simulink model "CollaborativeErgonomyControl"  (R2021b)
settings: Solver=FixedStepAuto  StartTime=0.0  StopTime=Config.SIMULATION_TIME  FixedStep=Config.tStep  RelTol=1e-3
InitFcn:
  | %% initialize the simulation
  | cd(fileparts(which(bdroot)));
  | initCollaborativeErgonomyControl;
StopFcn:
  | %% stop the simulation
  | cd(fileparts(which(bdroot)));
  | stopCollaborativeErgonomyControl;
values from neighbouring files (symbols this model uses):
  ConfigRobot1 = ConfigRobot    [initCollaborativeErgonomyControl.m]
  ConfigRobot2 = ConfigRobot    [initCollaborativeErgonomyControl.m]
undefined symbols (not defined in the file or in its folder): Config, ConfigObject
libraries: RobotStateLibrary x61, WBToolboxLibrary x40, MultiBodyLibrary x4, simulink x3
(part 1 of 2)
settings Model: NumberOfSteps=100  Creator=lorenzorapetti  LastModifiedBy=icub
settings SolverCC: AlgebraicLoopSolver=TrustRegion
settings DebuggingCC: SFMachineParentedDataDiag=warning

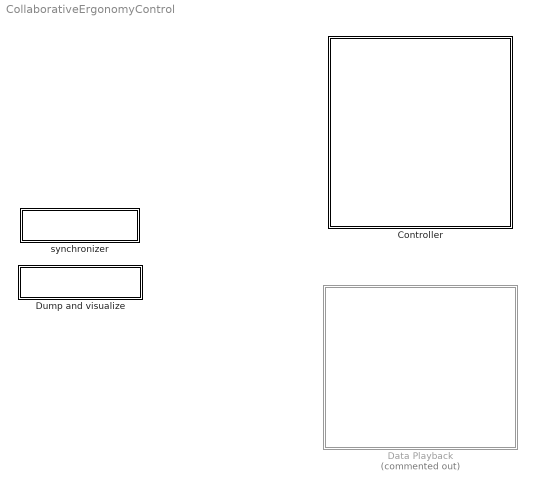
== system CollaborativeErgonomyControl ==
  Controller : Subsystem
  Data Playback : Subsystem  Commented=on
  Dump and visualize : Subsystem
      mask Display: disp('VISUALIZER')
  synchronizer : Subsystem
      mask Display: disp('SYNCHRONIZER')

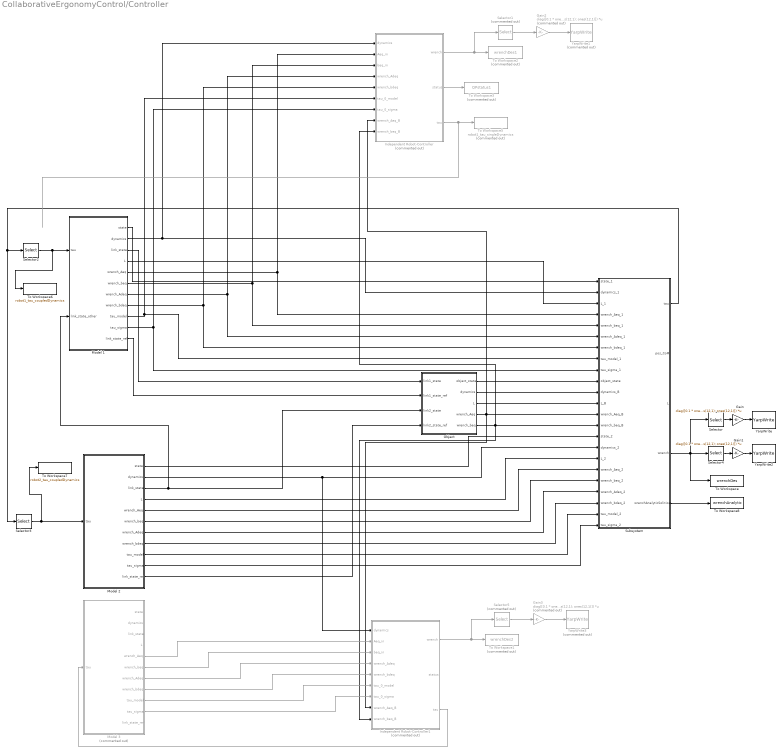
== system CollaborativeErgonomyControl/Controller ==
  Gain : Gain  Gain=diag([0.1 * ones(12,1); ones(12,1)])  Multiplication=Matrix(K*u) (u vector)
  Gain1 : Gain  Gain=diag([0.1 * ones(12,1); ones(12,1)])  Multiplication=Matrix(K*u) (u vector)
  Gain2 : Gain  Commented=on  Gain=diag([0.1 * ones(12,1); ones(12,1)])  Multiplication=Matrix(K*u) (u vector)
  Gain3 : Gain  Commented=on  Gain=diag([0.1 * ones(12,1); ones(12,1)])  Multiplication=Matrix(K*u) (u vector)
  Independent Robot-Controller : Subsystem  Commented=on
  Independent Robot-Controller1 : Subsystem  Commented=on
  Model 1 : Subsystem
  Model 2 : Subsystem
  Model 3 : Subsystem  Commented=on
  Object : Subsystem
  Selector : Selector  IndexOptions=Starting index (dialog)  Indices=1  OutputSizes=24
  Selector1 : Selector  Commented=on  IndexOptions=Starting index (dialog)  Indices=1  OutputSizes=24
  Selector2 : Selector  IndexOptions=Starting index (dialog)  Indices=1  OutputSizes=ConfigRobot1.ROBOT_DOF
  Selector3 : Selector  IndexOptions=Starting index (dialog)  Indices=1+ConfigRobot1.ROBOT_DOF  OutputSizes=ConfigRobot2.ROBOT_DOF
  Selector4 : Selector  IndexOptions=Starting index (dialog)  Indices=25  OutputSizes=24
  Selector5 : Selector  Commented=on  IndexOptions=Starting index (dialog)  Indices=1  OutputSizes=24
  Subsystem : Subsystem
  To Workspace : ToWorkspace  VariableName=wrenchDes  SaveFormat=Timeseries  SampleTime=-1
  To Workspace1 : ToWorkspace  Commented=on  VariableName=wrenchDes2  SaveFormat=Timeseries  SampleTime=-1
  To Workspace2 : ToWorkspace  Commented=on  VariableName=wrenchDes1  SaveFormat=Timeseries  SampleTime=-1
  To Workspace3 : ToWorkspace  Commented=on  VariableName=QPstatus1  SaveFormat=Timeseries  SampleTime=-1
  To Workspace5 : ToWorkspace  Commented=on  VariableName=robot1_tau_singleDynamics  SaveFormat=Timeseries  SampleTime=-1
  To Workspace6 : ToWorkspace  VariableName=robot1_tau_coupledDynamics  SaveFormat=Timeseries  SampleTime=-1
  To Workspace7 : ToWorkspace  VariableName=robot2_tau_coupledDynamics  SaveFormat=Timeseries  SampleTime=-1
  To Workspace8 : ToWorkspace  VariableName=wrenchAnalytic  SaveFormat=Timeseries  SampleTime=-1
  YarpWrite : WBToolboxLibrary/Utilities/YarpWrite  portName='/collaborativeController/robot1/wrench:o'  autoconnect=off  errorOnConnection=on
      settings: SourceProductName=WholeBodyToolbox
  YarpWrite1 : WBToolboxLibrary/Utilities/YarpWrite  Commented=on  portName='/collaborativeController/robot1/singleWrench:o'  autoconnect=off  errorOnConnection=on
      settings: SourceProductName=WholeBodyToolbox
  YarpWrite2 : WBToolboxLibrary/Utilities/YarpWrite  portName='/collaborativeController/robot2/wrench:o'  autoconnect=off  errorOnConnection=on
      settings: SourceProductName=WholeBodyToolbox
  YarpWrite3 : WBToolboxLibrary/Utilities/YarpWrite  Commented=on  portName='/collaborativeController/robot2/singleWrench:o'  autoconnect=off  errorOnConnection=on
      settings: SourceProductName=WholeBodyToolbox
  wires:
  Model 1/11(link_state_ref) -> Object/2(link1_state_ref)
  Object/2(dynamics) -> Subsystem/11(dynamics_B)
  Object/1(object_state) -> Subsystem/10(object_state)
  Model 2/1(state) -> Subsystem/15(state_2)
  Model 1/8(wrench_bdeq) -> Independent Robot-Controller/5(wrench_bdeq), Subsystem/7(wrench_bdeq_1)
  Model 1/2(dynamics) -> Independent Robot-Controller/1(dynamics), Subsystem/2(dynamics_1)
  Model 2/11(link_state_ref) -> Object/4(link2_state_ref)
  Subsystem/1(tau) -> Selector3/1, Selector2/1
  Model 2/10(tau_sigma) -> Subsystem/23(tau_sigma_2)
  Model 1/1(state) -> Subsystem/1(state_1)
  Model 2/4(L) -> Subsystem/17(L_2)
  Object/5(wrench_beq) -> Independent Robot-Controller1/9(wrench_beq_B), Independent Robot-Controller/9(wrench_beq_B), Subsystem/14(wrench_beq_B)
  Model 1/4(L) -> Subsystem/3(L_1)
  Model 2/2(dynamics) -> Independent Robot-Controller1/1(dynamics), Subsystem/16(dynamics_2)
  Model 2/9(tau_model) -> Subsystem/22(tau_model_2)
  Model 2/6(wrench_beq) -> Subsystem/19(wrench_beq_2)
  Object/4(wrench_Aeq) -> Independent Robot-Controller1/8(wrench_Aeq_B), Independent Robot-Controller/8(wrench_Aeq_B), Subsystem/13(wrench_Aeq_B)
  Model 2/3(link_state) -> Model 1/2(link_state_other), Object/3(link2_state)
  Model 2/5(wrench_Aeq) -> Subsystem/18(wrench_Aeq_2)
  Model 2/7(wrench_Adeq) -> Subsystem/20(wrench_Adeq_2)
  Independent Robot-Controller/2(status) -> To Workspace3/1
  Model 1/3(link_state) -> Object/1(link1_state)
  Model 1/10(tau_sigma) -> Independent Robot-Controller/7(tau_0_sigma), Subsystem/9(tau_sigma_1)
  Model 2/8(wrench_bdeq) -> Subsystem/21(wrench_bdeq_2)
  Model 1/5(wrench_Aeq) -> Independent Robot-Controller/2(Aeq_in), Subsystem/4(wrench_Aeq_1)
  Model 1/7(wrench_Adeq) -> Independent Robot-Controller/4(wrench_Adeq), Subsystem/6(wrench_Adeq_1)
  Object/3(L) -> Subsystem/12(L_B)
  Model 1/6(wrench_beq) -> Independent Robot-Controller/3(beq_in), Subsystem/5(wrench_beq_1)
  Model 1/9(tau_model) -> Independent Robot-Controller/6(tau_0_model), Subsystem/8(tau_model_1)
  Independent Robot-Controller1/3(tau) -> Model 3/1(tau)
  Selector3/1 -> To Workspace7/1, Model 2/1(tau)
  Model 3/5(wrench_Aeq) -> Independent Robot-Controller1/2(Aeq_in)
  Model 3/6(wrench_beq) -> Independent Robot-Controller1/3(beq_in)
  Model 3/7(wrench_Adeq) -> Independent Robot-Controller1/4(wrench_Adeq)
  Model 3/8(wrench_bdeq) -> Independent Robot-Controller1/5(wrench_bdeq)
  Model 3/9(tau_model) -> Independent Robot-Controller1/6(tau_0_model)
  Model 3/10(tau_sigma) -> Independent Robot-Controller1/7(tau_0_sigma)
  Independent Robot-Controller/3(tau) -> To Workspace5/1
  Selector/1 -> Gain/1
  Independent Robot-Controller/1(wrench) -> Selector1/1, To Workspace2/1
  Subsystem/4(wrench) -> Selector4/1, To Workspace/1, Selector/1
  Gain/1 -> YarpWrite/1
  Selector4/1 -> Gain1/1
  Gain1/1 -> YarpWrite2/1
  Gain2/1 -> YarpWrite1/1
  Selector1/1 -> Gain2/1
  Subsystem/5(wrenchAnalyticSolition) -> To Workspace8/1
  Independent Robot-Controller1/1(wrench) -> Selector5/1, To Workspace1/1
  Selector5/1 -> Gain3/1
  Gain3/1 -> YarpWrite3/1
  Selector2/1 -> To Workspace6/1, Model 1/1(tau)

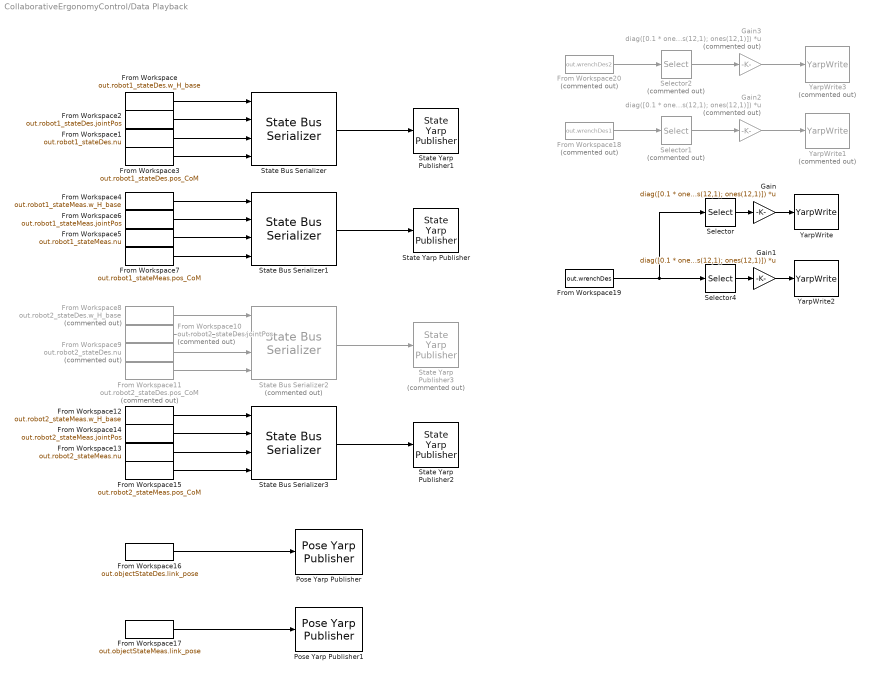
== system CollaborativeErgonomyControl/Data Playback ==
  From Workspace : FromWorkspace  VariableName=out.robot1_stateDes.w_H_base  OutputAfterFinalValue=Holding final value
  From Workspace1 : FromWorkspace  VariableName=out.robot1_stateDes.nu  OutputAfterFinalValue=Holding final value
  From Workspace10 : FromWorkspace  Commented=on  VariableName=out.robot2_stateDes.jointPos  OutputAfterFinalValue=Holding final value
  From Workspace11 : FromWorkspace  Commented=on  VariableName=out.robot2_stateDes.pos_CoM  OutputAfterFinalValue=Holding final value
  From Workspace12 : FromWorkspace  VariableName=out.robot2_stateMeas.w_H_base  OutputAfterFinalValue=Holding final value
  From Workspace13 : FromWorkspace  VariableName=out.robot2_stateMeas.nu  OutputAfterFinalValue=Holding final value
  From Workspace14 : FromWorkspace  VariableName=out.robot2_stateMeas.jointPos  OutputAfterFinalValue=Holding final value
  From Workspace15 : FromWorkspace  VariableName=out.robot2_stateMeas.pos_CoM  OutputAfterFinalValue=Holding final value
  From Workspace16 : FromWorkspace  VariableName=out.objectStateDes.link_pose  OutputAfterFinalValue=Holding final value
  From Workspace17 : FromWorkspace  VariableName=out.objectStateMeas.link_pose  OutputAfterFinalValue=Holding final value
  From Workspace18 : FromWorkspace  Commented=on  VariableName=out.wrenchDes1  OutputAfterFinalValue=Holding final value
  From Workspace19 : FromWorkspace  VariableName=out.wrenchDes  OutputAfterFinalValue=Holding final value
  From Workspace2 : FromWorkspace  VariableName=out.robot1_stateDes.jointPos  OutputAfterFinalValue=Holding final value
  From Workspace20 : FromWorkspace  Commented=on  VariableName=out.wrenchDes2  OutputAfterFinalValue=Holding final value
  From Workspace3 : FromWorkspace  VariableName=out.robot1_stateDes.pos_CoM  OutputAfterFinalValue=Holding final value
  From Workspace4 : FromWorkspace  VariableName=out.robot1_stateMeas.w_H_base  OutputAfterFinalValue=Holding final value
  From Workspace5 : FromWorkspace  VariableName=out.robot1_stateMeas.nu  OutputAfterFinalValue=Holding final value
  From Workspace6 : FromWorkspace  VariableName=out.robot1_stateMeas.jointPos  OutputAfterFinalValue=Holding final value
  From Workspace7 : FromWorkspace  VariableName=out.robot1_stateMeas.pos_CoM  OutputAfterFinalValue=Holding final value
  From Workspace8 : FromWorkspace  Commented=on  VariableName=out.robot2_stateDes.w_H_base  OutputAfterFinalValue=Holding final value
  From Workspace9 : FromWorkspace  Commented=on  VariableName=out.robot2_stateDes.nu  OutputAfterFinalValue=Holding final value
  Gain : Gain  Gain=diag([0.1 * ones(12,1); ones(12,1)])  Multiplication=Matrix(K*u) (u vector)
  Gain1 : Gain  Gain=diag([0.1 * ones(12,1); ones(12,1)])  Multiplication=Matrix(K*u) (u vector)
  Gain2 : Gain  Commented=on  Gain=diag([0.1 * ones(12,1); ones(12,1)])  Multiplication=Matrix(K*u) (u vector)
  Gain3 : Gain  Commented=on  Gain=diag([0.1 * ones(12,1); ones(12,1)])  Multiplication=Matrix(K*u) (u vector)
  Pose Yarp Publisher : RobotStateLibrary/Pose Yarp Publisher  portName='/collaborativeController/boxRef/basePose:o'
      settings: SourceProductName=robot-state-library
  Pose Yarp Publisher1 : RobotStateLibrary/Pose Yarp Publisher  portName='/collaborativeController/box/basePose:o'
      settings: SourceProductName=robot-state-library
  Selector : Selector  IndexOptions=Starting index (dialog)  Indices=1  OutputSizes=24
  Selector1 : Selector  Commented=on  IndexOptions=Starting index (dialog)  Indices=1  OutputSizes=24
  Selector2 : Selector  Commented=on  IndexOptions=Starting index (dialog)  Indices=1  OutputSizes=24
  Selector4 : Selector  IndexOptions=Starting index (dialog)  Indices=25  OutputSizes=24
  State Bus Serializer : RobotStateLibrary/State Bus Serializer  SystemSampleTime=-1  VariantActivationTime=update diagram  Latency=0  AutoFrameSizeCalculation=off
      settings: SourceProductName=robot-state-library
  State Bus Serializer1 : RobotStateLibrary/State Bus Serializer  SystemSampleTime=-1  VariantActivationTime=update diagram  Latency=0  AutoFrameSizeCalculation=off
      settings: SourceProductName=robot-state-library
  State Bus Serializer2 : RobotStateLibrary/State Bus Serializer  Commented=on  SystemSampleTime=-1  VariantActivationTime=update diagram  Latency=0  AutoFrameSizeCalculation=off
      settings: SourceProductName=robot-state-library
  State Bus Serializer3 : RobotStateLibrary/State Bus Serializer  SystemSampleTime=-1  VariantActivationTime=update diagram  Latency=0  AutoFrameSizeCalculation=off
      settings: SourceProductName=robot-state-library
  State Yarp Publisher : RobotStateLibrary/State Yarp Publisher  basePosePortName='/collaborativeController/robot1/basePose:o'  jointPosPortName='/collaborativeController/robot1/jointPosition:o'  nuPortName='/collaborativeController/robot1/stateVelocity:o'  posCoMPortName='/collaborativeController/robot1/CoMPosition:o'
      settings: SourceProductName=robot-state-library
  State Yarp Publisher1 : RobotStateLibrary/State Yarp Publisher  basePosePortName='/collaborativeController/robot1Ref/basePose:o'  jointPosPortName='/collaborativeController/robot1Ref/jointPosition:o'  nuPortName='/collaborativeController/robot1Ref/stateVelocity:o'  posCoMPortName='/collaborativeController/robot1Ref/CoMPosition:o'
      settings: SourceProductName=robot-state-library
  State Yarp Publisher2 : RobotStateLibrary/State Yarp Publisher  basePosePortName='/collaborativeController/robot2/basePose:o'  jointPosPortName='/collaborativeController/robot2/jointPosition:o'  nuPortName='/collaborativeController/robot2/stateVelocity:o'  posCoMPortName='/collaborativeController/robot2/CoMPosition:o'
      settings: SourceProductName=robot-state-library
  State Yarp Publisher3 : RobotStateLibrary/State Yarp Publisher  Commented=on  basePosePortName='/collaborativeController/robot2Ref/basePose:o'  jointPosPortName='/collaborativeController/robot2Ref/jointPosition:o'  nuPortName='/collaborativeController/robot2Ref/stateVelocity:o'  posCoMPortName='/collaborativeController/robot2Ref/CoMPosition:o'
      settings: SourceProductName=robot-state-library
  YarpWrite : WBToolboxLibrary/Utilities/YarpWrite  portName='/collaborativeController/robot1/wrench:o'  autoconnect=off  errorOnConnection=on
      settings: SourceProductName=WholeBodyToolbox
  YarpWrite1 : WBToolboxLibrary/Utilities/YarpWrite  Commented=on  portName='/collaborativeController/robot1/singleWrench:o'  autoconnect=off  errorOnConnection=on
      settings: SourceProductName=WholeBodyToolbox
  YarpWrite2 : WBToolboxLibrary/Utilities/YarpWrite  portName='/collaborativeController/robot2/wrench:o'  autoconnect=off  errorOnConnection=on
      settings: SourceProductName=WholeBodyToolbox
  YarpWrite3 : WBToolboxLibrary/Utilities/YarpWrite  Commented=on  portName='/collaborativeController/robot2/singleWrench:o'  autoconnect=off  errorOnConnection=on
      settings: SourceProductName=WholeBodyToolbox
  wires:
  From Workspace3/1 -> State Bus Serializer/4
  State Bus Serializer/1 -> State Yarp Publisher1/1
  From Workspace2/1 -> State Bus Serializer/2
  From Workspace4/1 -> State Bus Serializer1/1
  From Workspace7/1 -> State Bus Serializer1/4
  From Workspace1/1 -> State Bus Serializer/3
  From Workspace6/1 -> State Bus Serializer1/2
  State Bus Serializer1/1 -> State Yarp Publisher/1
  From Workspace5/1 -> State Bus Serializer1/3
  From Workspace/1 -> State Bus Serializer/1
  From Workspace15/1 -> State Bus Serializer3/4
  From Workspace12/1 -> State Bus Serializer3/1
  State Bus Serializer2/1 -> State Yarp Publisher3/1
  From Workspace8/1 -> State Bus Serializer2/1
  From Workspace14/1 -> State Bus Serializer3/2
  From Workspace10/1 -> State Bus Serializer2/2
  State Bus Serializer3/1 -> State Yarp Publisher2/1
  From Workspace11/1 -> State Bus Serializer2/4
  From Workspace13/1 -> State Bus Serializer3/3
  From Workspace9/1 -> State Bus Serializer2/3
  From Workspace16/1 -> Pose Yarp Publisher/1
  From Workspace17/1 -> Pose Yarp Publisher1/1
  Gain2/1 -> YarpWrite1/1
  Selector1/1 -> Gain2/1
  From Workspace18/1 -> Selector1/1
  Gain1/1 -> YarpWrite2/1
  Selector/1 -> Gain/1
  From Workspace19/1 -> Selector4/1, Selector/1
  Selector4/1 -> Gain1/1
  Gain/1 -> YarpWrite/1
  From Workspace20/1 -> Selector2/1
  Gain3/1 -> YarpWrite3/1
  Selector2/1 -> Gain3/1

== system CollaborativeErgonomyControl/Dump and visualize ==
  Clock : Clock
  TIME_SCOPE : Constant  Value=Config.Scopes.TIME_SCOPE
  Time Scope : Subsystem
  wires:
  TIME_SCOPE/1 -> Time Scope/Enable
  [yarp_time] -> Time Scope/1(yarp_time)
  Clock/1 -> Time Scope/2(simulink_time)

== system CollaborativeErgonomyControl/synchronizer ==
  GAZEBO_SYNCHRONIZER : Subsystem
  Logical Operator : Logic  Operator=NOT  AllPortsSameDT=off  OutDataTypeStr=boolean
  "ON_GAZEBO " : Constant  Value=Config.ON_GAZEBO
  REAL_TIME_SYNC : Subsystem
  To Workspace : ToWorkspace  VariableName=yarp_time  SaveFormat=Structure With Time  SampleTime=-1
  Yarp Clock : WBToolboxLibrary/Utilities/Yarp Clock
      settings: SourceProductName=WholeBodyToolbox
  tag scope: yarp_time=global
  wires:
  Logical Operator/1 -> REAL_TIME_SYNC/Enable
  "ON_GAZEBO "/1 -> GAZEBO_SYNCHRONIZER/Enable, Logical Operator/1
  Yarp Clock/1 -> [yarp_time], To Workspace/1

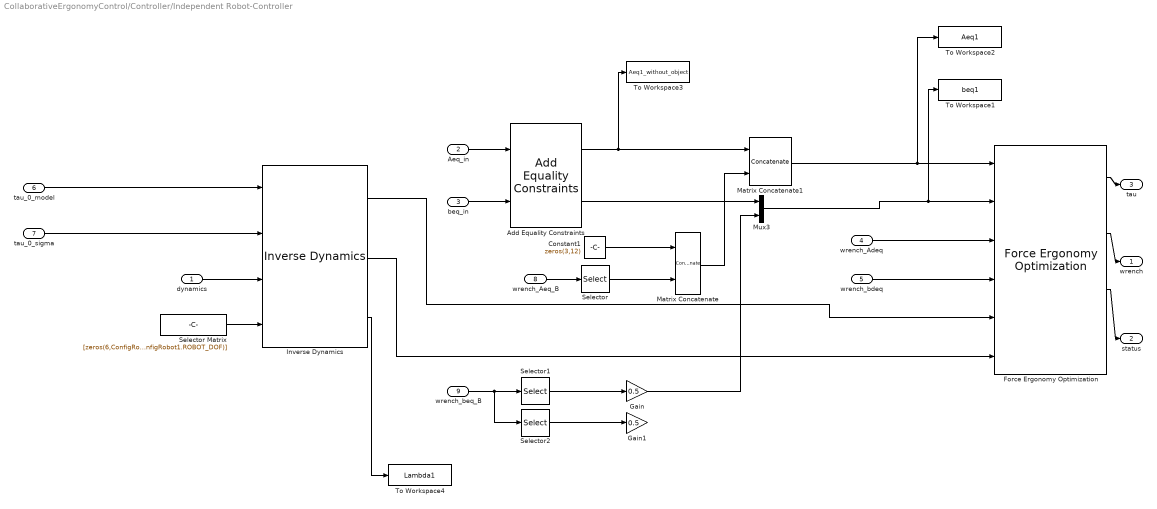
== system CollaborativeErgonomyControl/Controller/Independent Robot-Controller ==
  dynamics : Inport
  Aeq_in : Inport  Port=2
  beq_in : Inport  Port=3
  wrench_Adeq : Inport  Port=4
  wrench_bdeq : Inport  Port=5
  tau_0_model : Inport  Port=6
  tau_0_sigma : Inport  Port=7
  wrench_Aeq_B : Inport  Port=8
  wrench_beq_B : Inport  Port=9
  Add Equality Constraints : RobotStateLibrary/Add Equality Constraints  Aeq_add=ConfigRobot1.wrench_Aeq_const  beq_add=ConfigRobot1.wrench_beq_const
      settings: SourceProductName=robot-state-library
  Constant1 : Constant  Value=zeros(3,12)
  Force Ergonomy Optimization : RobotStateLibrary/Force Ergonomy Optimization  InvTol=ConfigRobot1.Reg.AInvTol  regularizationHessian=ConfigRobot1.Reg.Hessian  minimizationWeight=ConfigRobot1.Gains.tauMinimization
      settings: SourceProductName=robot-state-library
  Gain : Gain  Gain=0.5
  Gain1 : Gain  Gain=0.5
  Inverse Dynamics : RobotStateLibrary/Inverse Dynamics  Reg=ConfigRobot1.Reg  fixedLinkVelcityComponents=ConfigRobot1.fixedLinkVelcityComponents
      settings: SourceProductName=robot-state-library
  Matrix Concatenate : Concatenate  Mode=Multidimensional array  ConcatenateDimension=2
  Matrix Concatenate1 : Concatenate  Mode=Multidimensional array
  Mux3 : Mux  Inputs=2
  Selector : Selector  NumberOfDimensions=2  InputPortWidth=3  IndexOptions=Starting index (dialog),Starting index (dialog)  Indices=1,1  OutputSizes=3,12
  Selector Matrix : Constant  Value=[zeros(6,ConfigRobot1.ROBOT_DOF); eye(ConfigRobot1.ROBOT_DOF)]
  Selector1 : Selector  InputPortWidth=6  IndexOptions=Starting index (dialog)  Indices=1  OutputSizes=3
  Selector2 : Selector  InputPortWidth=6  IndexOptions=Starting index (dialog)  Indices=4  OutputSizes=3
  To Workspace1 : ToWorkspace  VariableName=beq1  SaveFormat=Timeseries  SampleTime=-1
  To Workspace2 : ToWorkspace  VariableName=Aeq1  SaveFormat=Timeseries  SampleTime=-1
  To Workspace3 : ToWorkspace  VariableName=Aeq1_without_object  SaveFormat=Timeseries  SampleTime=-1
  To Workspace4 : ToWorkspace  VariableName=Lambda1  SaveFormat=Timeseries  SampleTime=-1
  wrench : Outport
  status : Outport  Port=2
  tau : Outport  Port=3
  wires:
  wrench_Aeq_B/1 -> Selector/1
  Add Equality Constraints/2 -> Mux3/1
  Constant1/1 -> Matrix Concatenate/1
  wrench_bdeq/1 -> Force Ergonomy Optimization/4
  dynamics/1 -> Inverse Dynamics/3
  Inverse Dynamics/2 -> Force Ergonomy Optimization/6
  wrench_Adeq/1 -> Force Ergonomy Optimization/3
  tau_0_sigma/1 -> Inverse Dynamics/2
  Inverse Dynamics/1 -> Force Ergonomy Optimization/5
  Aeq_in/1 -> Add Equality Constraints/1
  beq_in/1 -> Add Equality Constraints/2
  Force Ergonomy Optimization/3 -> status/1
  Selector/1 -> Matrix Concatenate/2
  Gain/1 -> Mux3/2
  Matrix Concatenate/1 -> Matrix Concatenate1/2
  tau_0_model/1 -> Inverse Dynamics/1
  Force Ergonomy Optimization/2 -> wrench/1
  Force Ergonomy Optimization/1 -> tau/1
  Selector Matrix/1 -> Inverse Dynamics/4
  Add Equality Constraints/1 -> To Workspace3/1, Matrix Concatenate1/1
  wrench_beq_B/1 -> Selector2/1, Selector1/1
  Selector1/1 -> Gain/1
  Selector2/1 -> Gain1/1
  Matrix Concatenate1/1 -> To Workspace2/1, Force Ergonomy Optimization/1
  Mux3/1 -> To Workspace1/1, Force Ergonomy Optimization/2
  Inverse Dynamics/3 -> To Workspace4/1

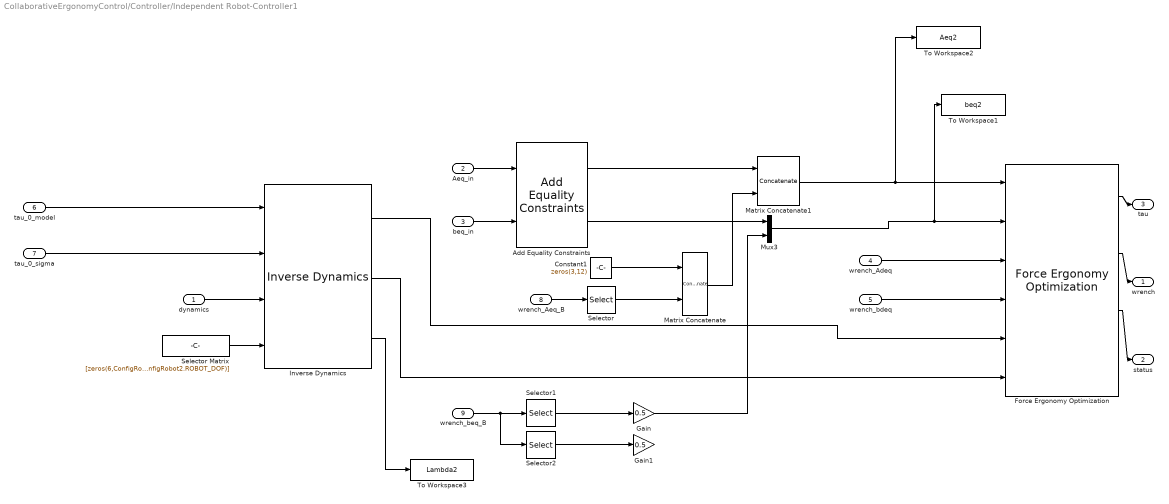
== system CollaborativeErgonomyControl/Controller/Independent Robot-Controller1 ==
  dynamics : Inport
  Aeq_in : Inport  Port=2
  beq_in : Inport  Port=3
  wrench_Adeq : Inport  Port=4
  wrench_bdeq : Inport  Port=5
  tau_0_model : Inport  Port=6
  tau_0_sigma : Inport  Port=7
  wrench_Aeq_B : Inport  Port=8
  wrench_beq_B : Inport  Port=9
  Add Equality Constraints : RobotStateLibrary/Add Equality Constraints  Aeq_add=ConfigRobot2.wrench_Aeq_const  beq_add=ConfigRobot2.wrench_beq_const
      settings: SourceProductName=robot-state-library
  Constant1 : Constant  Value=zeros(3,12)
  Force Ergonomy Optimization : RobotStateLibrary/Force Ergonomy Optimization  InvTol=ConfigRobot2.Reg.AInvTol  regularizationHessian=ConfigRobot2.Reg.Hessian  minimizationWeight=ConfigRobot2.Gains.tauMinimization
      settings: SourceProductName=robot-state-library
  Gain : Gain  Gain=0.5
  Gain1 : Gain  Gain=0.5
  Inverse Dynamics : RobotStateLibrary/Inverse Dynamics  Reg=ConfigRobot2.Reg  fixedLinkVelcityComponents=ConfigRobot2.fixedLinkVelcityComponents
      settings: SourceProductName=robot-state-library
  Matrix Concatenate : Concatenate  Mode=Multidimensional array  ConcatenateDimension=2
  Matrix Concatenate1 : Concatenate  Mode=Multidimensional array
  Mux3 : Mux  Inputs=2
  Selector : Selector  NumberOfDimensions=2  InputPortWidth=3  IndexOptions=Starting index (dialog),Starting index (dialog)  Indices=1,13  OutputSizes=3,12
  Selector Matrix : Constant  Value=[zeros(6,ConfigRobot2.ROBOT_DOF); eye(ConfigRobot2.ROBOT_DOF)]
  Selector1 : Selector  InputPortWidth=6  IndexOptions=Starting index (dialog)  Indices=1  OutputSizes=3
  Selector2 : Selector  InputPortWidth=6  IndexOptions=Starting index (dialog)  Indices=4  OutputSizes=3
  To Workspace1 : ToWorkspace  VariableName=beq2  SaveFormat=Timeseries  SampleTime=-1
  To Workspace2 : ToWorkspace  VariableName=Aeq2  SaveFormat=Timeseries  SampleTime=-1
  To Workspace3 : ToWorkspace  VariableName=Lambda2  SaveFormat=Timeseries  SampleTime=-1
  wrench : Outport
  status : Outport  Port=2
  tau : Outport  Port=3
  wires:
  wrench_Aeq_B/1 -> Selector/1
  Add Equality Constraints/2 -> Mux3/1
  Constant1/1 -> Matrix Concatenate/1
  wrench_bdeq/1 -> Force Ergonomy Optimization/4
  dynamics/1 -> Inverse Dynamics/3
  Inverse Dynamics/2 -> Force Ergonomy Optimization/6
  wrench_Adeq/1 -> Force Ergonomy Optimization/3
  tau_0_sigma/1 -> Inverse Dynamics/2
  Inverse Dynamics/1 -> Force Ergonomy Optimization/5
  Aeq_in/1 -> Add Equality Constraints/1
  beq_in/1 -> Add Equality Constraints/2
  Force Ergonomy Optimization/3 -> status/1
  Selector/1 -> Matrix Concatenate/2
  Gain/1 -> Mux3/2
  Matrix Concatenate/1 -> Matrix Concatenate1/2
  tau_0_model/1 -> Inverse Dynamics/1
  Force Ergonomy Optimization/2 -> wrench/1
  Force Ergonomy Optimization/1 -> tau/1
  Selector Matrix/1 -> Inverse Dynamics/4
  Add Equality Constraints/1 -> Matrix Concatenate1/1
  wrench_beq_B/1 -> Selector2/1, Selector1/1
  Selector1/1 -> Gain/1
  Selector2/1 -> Gain1/1
  Matrix Concatenate1/1 -> To Workspace2/1, Force Ergonomy Optimization/1
  Mux3/1 -> To Workspace1/1, Force Ergonomy Optimization/2
  Inverse Dynamics/3 -> To Workspace3/1

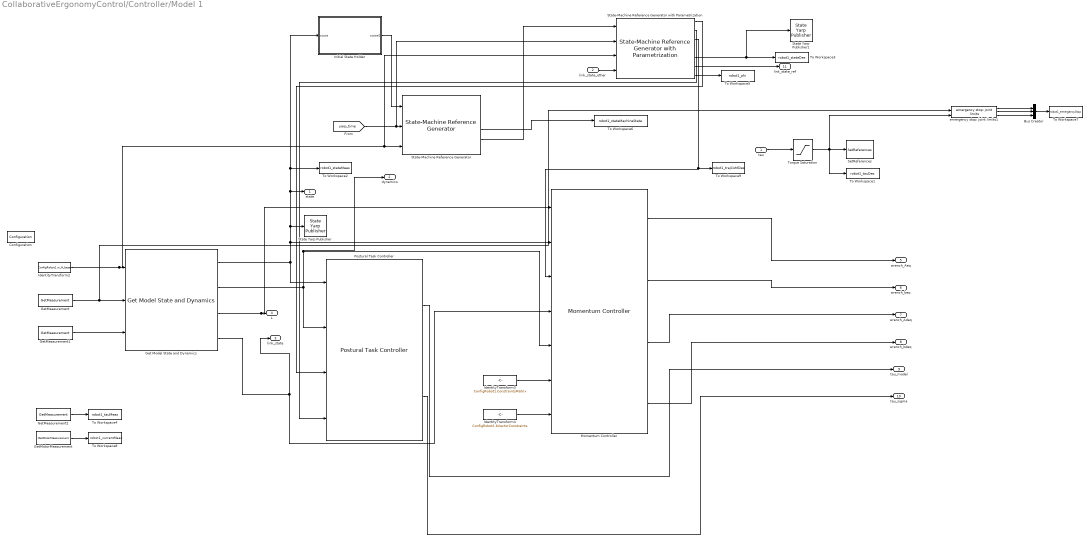
== system CollaborativeErgonomyControl/Controller/Model 1 ==
  tau : Inport
  link_state_other : Inport  Port=2
  Bus Creator : BusCreator  Inputs=3
  Configuration : WBToolboxLibrary/Utilities/Configuration  ConfigSource=Workspace  ConfigObject='WBTConfigRobot_1'
      settings: SourceProductName=WholeBodyToolbox
  Get Model State and Dynamics : RobotStateLibrary/Get Model State and Dynamics  nDoF=ConfigRobot1.ROBOT_DOF  regularization=0.1  contactFrame1Name=ConfigRobot1.Frames.LEFT_FOOT  contactFrame2Name=ConfigRobot1.Frames.RIGHT_FOOT  frame1=ConfigRobot1.Frames.LEFT_FOOT  frame2=ConfigRobot1.Frames.RIGHT_FOOT  frame3=ConfigRobot1.Frames.LEFT_HAND  frame4=ConfigRobot1.Frames.RIGHT_HAND
      settings: SourceProductName=robot-state-library
  GetMeasurement : WBToolboxLibrary/States/GetMeasurement  measuredType=Joints Position
      settings: SourceProductName=WholeBodyToolbox
  GetMeasurement1 : WBToolboxLibrary/States/GetMeasurement  measuredType=Joints Velocity
      settings: SourceProductName=WholeBodyToolbox
  GetMeasurement2 : WBToolboxLibrary/States/GetMeasurement  measuredType=Joints Torque
      settings: SourceProductName=WholeBodyToolbox
  GetMotorMeasurement : WBToolboxLibrary/States/GetMotorMeasurement  measuredType=Motor Current
      settings: SourceProductName=WholeBodyToolbox
  IdentityTransform2 : Constant  Value=ConfigRobot1.w_H_base
  IdentityTransform3 : Constant  Value=ConfigRobot1.ConstraintsMatrix
  IdentityTransform4 : Constant  Value=ConfigRobot1.bVectorConstraints
  Initial State Holder : Subsystem
  Momentum Controller : RobotStateLibrary/Momentum Controller  GainMomentum=ConfigRobot1.Gains.GainMomentum  linksUseConstraintMatrix=ConfigRobot1.linksUseConstraintMatrix
      settings: SourceProductName=robot-state-library
  Postural Task Controller : RobotStateLibrary/Postural Task Controller  GainPostural=ConfigRobot1.Gains.GainPostural
      settings: SourceProductName=robot-state-library
  SetReferences : WBToolboxLibrary/Actuators/SetReferences  controlType=Torque  refSpeed=10*(pi/180)  refAcceleration=1000000*(pi/180)
      settings: SourceProductName=WholeBodyToolbox
  State Yarp Publisher : RobotStateLibrary/State Yarp Publisher  basePosePortName='/collaborativeController/robot1/basePose:o'  jointPosPortName='/collaborativeController/robot1/jointPosition:o'  nuPortName='/collaborativeController/robot1/stateVelocity:o'  posCoMPortName='/collaborativeController/robot1/CoMPosition:o'
      settings: SourceProductName=robot-state-library
  State Yarp Publisher1 : RobotStateLibrary/State Yarp Publisher  basePosePortName='/collaborativeController/robot1Ref/basePose:o'  jointPosPortName='/collaborativeController/robot1Ref/jointPosition:o'  nuPortName='/collaborativeController/robot1Ref/stateVelocity:o'  posCoMPortName='/collaborativeController/robot1Ref/CoMPosition:o'
      settings: SourceProductName=robot-state-library
  State-Machine Reference Generator : RobotStateLibrary/State-Machine Reference Generator  configStateMachine=ConfigRobot1.StateMachine  sampleTime=Config.tStep  frameName1=ConfigRobot1.Frames.LEFT_FOOT  frameName2=ConfigRobot1.Frames.RIGHT_FOOT  regularization=0.1  nDoF=ConfigRobot1.ROBOT_DOF  frame1=ConfigRobot1.Frames.LEFT_FOOT  frame2=ConfigRobot1.Frames.RIGHT_FOOT  frame3=ConfigRobot1.Frames.LEFT_HAND  frame4=ConfigRobot1.Frames.RIGHT_HAND
      settings: SourceProductName=robot-state-library
  State-Machine Reference Generator with Parametrization : RobotStateLibrary/State-Machine Reference Generator with Parametrization  configStateMachine=ConfigRobot1.StateMachine  frameName1=ConfigRobot1.Frames.LEFT_FOOT  frameName2=ConfigRobot1.Frames.RIGHT_FOOT  regularization=0.1  nDoF=ConfigRobot1.ROBOT_DOF  frame1=ConfigRobot1.Frames.LEFT_FOOT  frame2=ConfigRobot1.Frames.RIGHT_FOOT  frame3=ConfigRobot1.Frames.LEFT_HAND  frame4=ConfigRobot1.Frames.RIGHT_HAND  settlingTime=Config.com_minJerk_settlingTime  sampleTime=Config.tStep
      link override Constant: Value=1
      settings: SourceProductName=robot-state-library
  To Workspace1 : ToWorkspace  VariableName=robot1_tauDes  SaveFormat=Timeseries  SampleTime=-1
  To Workspace2 : ToWorkspace  VariableName=robot1_stateMeas  SaveFormat=Timeseries  SampleTime=-1
  To Workspace3 : ToWorkspace  VariableName=robot1_stateDes  SaveFormat=Timeseries  SampleTime=-1
  To Workspace4 : ToWorkspace  VariableName=robot1_tauMeas  SaveFormat=Timeseries  SampleTime=-1
  To Workspace5 : ToWorkspace  VariableName=robot1_phi  SaveFormat=Timeseries  SampleTime=-1
  To Workspace6 : ToWorkspace  VariableName=robot1_stateMachineState  SaveFormat=Timeseries  SampleTime=-1
  To Workspace7 : ToWorkspace  VariableName=robot1_emergencyStop  SaveFormat=Timeseries  SampleTime=-1
  To Workspace8 : ToWorkspace  VariableName=robot1_currentMeas  SaveFormat=Timeseries  SampleTime=-1
  To Workspace9 : ToWorkspace  VariableName=robot1_trajCoMDes  SaveFormat=Timeseries  SampleTime=-1
  Torque Saturation : Saturate  UpperLimit=ConfigRobot1.Safety.torqueSaturation  LowerLimit=-ConfigRobot1.Safety.torqueSaturation
  emergency stop: joint limits1 : RobotStateLibrary/emergency stop: joint limits  Safety=ConfigRobot1.Safety
      settings: SourceProductName=robot-state-library
  state : Outport
  dynamics : Outport  Port=2
  link_state : Outport  Port=3
  L : Outport  Port=4
  wrench_Aeq : Outport  Port=5
  wrench_beq : Outport  Port=6
  wrench_Adeq : Outport  Port=7
  wrench_bdeq : Outport  Port=8
  tau_model : Outport  Port=9
  tau_sigma : Outport  Port=10
  link_state_ref : Outport  Port=11
  wires:
  GetMeasurement/1 -> emergency stop: joint limits1/1, Get Model State and Dynamics/2
  GetMeasurement1/1 -> Get Model State and Dynamics/3
  IdentityTransform2/1 -> State-Machine Reference Generator with Parametrization/3, State-Machine Reference Generator/3, Get Model State and Dynamics/1
  Get Model State and Dynamics/3 -> Momentum Controller/1, L/1
  [yarp_time] -> State-Machine Reference Generator with Parametrization/2, State-Machine Reference Generator/2
  State-Machine Reference Generator/5 -> State-Machine Reference Generator with Parametrization/1
  Get Model State and Dynamics/1 -> Postural Task Controller/1, Momentum Controller/2, To Workspace2/1, Initial State Holder/1(state), state/1, State Yarp Publisher/1
  Initial State Holder/1(state0) -> State-Machine Reference Generator/1
  Get Model State and Dynamics/4 -> link_state/1, Momentum Controller/4
  Get Model State and Dynamics/2 -> Postural Task Controller/2, Momentum Controller/5, dynamics/1
  Momentum Controller/3 -> wrench_Adeq/1
  Momentum Controller/4 -> wrench_bdeq/1
  Postural Task Controller/1 -> tau_model/1
  Postural Task Controller/2 -> tau_sigma/1
  Momentum Controller/1 -> wrench_Aeq/1
  Momentum Controller/2 -> wrench_beq/1
  tau/1 -> Torque Saturation/1
  emergency stop: joint limits1/2 -> Bus Creator/2
  Bus Creator/1 -> To Workspace7/1
  emergency stop: joint limits1/3 -> Bus Creator/3
  emergency stop: joint limits1/1 -> Bus Creator/1
  State-Machine Reference Generator/4 -> To Workspace6/1
  GetMeasurement2/1 -> To Workspace4/1
  Torque Saturation/1 -> emergency stop: joint limits1/2, To Workspace1/1, SetReferences/1
  link_state_other/1 -> State-Machine Reference Generator with Parametrization/4
  State-Machine Reference Generator with Parametrization/1 -> Postural Task Controller/3
  State-Machine Reference Generator with Parametrization/6 -> link_state_ref/1
  State-Machine Reference Generator with Parametrization/7 -> To Workspace5/1
  State-Machine Reference Generator with Parametrization/5 -> To Workspace3/1, State Yarp Publisher1/1
  GetMotorMeasurement/1 -> To Workspace8/1
  State-Machine Reference Generator with Parametrization/2 -> Postural Task Controller/4
  State-Machine Reference Generator with Parametrization/3 -> Momentum Controller/3, To Workspace9/1
  IdentityTransform3/1 -> Momentum Controller/6
  IdentityTransform4/1 -> Momentum Controller/7

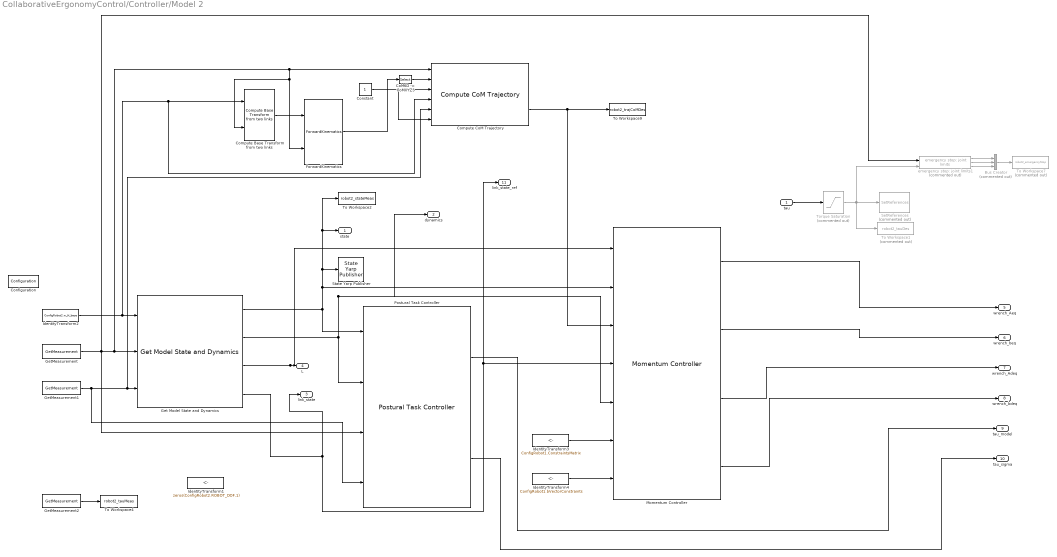
== system CollaborativeErgonomyControl/Controller/Model 2 ==
  tau : Inport
  Bus Creator : BusCreator  Commented=on  Inputs=3
  "CoM6D -> CoMXYZ3" : Selector  NumberOfDimensions=2  InputPortWidth=7  IndexOptions=Index vector (dialog),Index vector (dialog)  Indices=[1 2 3],[4]  OutputSizes=1,1
  Compute Base Transform from two links : RobotStateLibrary/Compute Base Transform from two links  frameName1=ConfigRobot2.Frames.LEFT_FOOT  frameName2=ConfigRobot2.Frames.RIGHT_FOOT
      settings: SourceProductName=robot-state-library
  Compute CoM Trajectory : RobotStateLibrary/Compute CoM Trajectory  frameName1=ConfigRobot2.Frames.LEFT_FOOT  frameName2=ConfigRobot2.Frames.RIGHT_FOOT  regularization=0.1
      settings: SourceProductName=robot-state-library
  Configuration : WBToolboxLibrary/Utilities/Configuration  ConfigSource=Workspace  ConfigObject='WBTConfigRobot_2'
      settings: SourceProductName=WholeBodyToolbox
  Constant : Constant
  ForwardKinematics : WBToolboxLibrary/Model/Kinematics/ForwardKinematics  frameName='com'
      settings: SourceProductName=WholeBodyToolbox
  Get Model State and Dynamics : RobotStateLibrary/Get Model State and Dynamics  nDoF=ConfigRobot2.ROBOT_DOF  regularization=0.1  contactFrame1Name=ConfigRobot2.Frames.LEFT_FOOT  contactFrame2Name=ConfigRobot2.Frames.RIGHT_FOOT  frame1=ConfigRobot2.Frames.LEFT_FOOT  frame2=ConfigRobot2.Frames.RIGHT_FOOT  frame3=ConfigRobot2.Frames.LEFT_HAND  frame4=ConfigRobot2.Frames.RIGHT_HAND
      settings: SourceProductName=robot-state-library
  GetMeasurement : WBToolboxLibrary/States/GetMeasurement  measuredType=Joints Position
      settings: SourceProductName=WholeBodyToolbox
  GetMeasurement1 : WBToolboxLibrary/States/GetMeasurement  measuredType=Joints Velocity
      settings: SourceProductName=WholeBodyToolbox
  GetMeasurement2 : WBToolboxLibrary/States/GetMeasurement  measuredType=Joints Torque
      settings: SourceProductName=WholeBodyToolbox
  IdentityTransform1 : Constant  Value=zeros(ConfigRobot2.ROBOT_DOF,1)
  IdentityTransform2 : Constant  Value=ConfigRobot2.w_H_base
  IdentityTransform3 : Constant  Value=ConfigRobot1.ConstraintsMatrix
  IdentityTransform4 : Constant  Value=ConfigRobot1.bVectorConstraints
  Momentum Controller : RobotStateLibrary/Momentum Controller  GainMomentum=GainMomentumDummy  linksUseConstraintMatrix=ConfigRobot2.linksUseConstraintMatrix
      settings: SourceProductName=robot-state-library
  Postural Task Controller : RobotStateLibrary/Postural Task Controller  GainPostural=GainPosturalDummy
      settings: SourceProductName=robot-state-library
  SetReferences : WBToolboxLibrary/Actuators/SetReferences  Commented=on  controlType=Torque  refSpeed=10*(pi/180)  refAcceleration=1000000*(pi/180)
      settings: SourceProductName=WholeBodyToolbox
  State Yarp Publisher : RobotStateLibrary/State Yarp Publisher  basePosePortName='/collaborativeController/robot2/basePose:o'  jointPosPortName='/collaborativeController/robot2/jointPosition:o'  nuPortName='/collaborativeController/robot2/stateVelocity:o'  posCoMPortName='/collaborativeController/robot2/CoMPosition:o'
      settings: SourceProductName=robot-state-library
  To Workspace1 : ToWorkspace  Commented=on  VariableName=robot2_tauDes  SaveFormat=Timeseries  SampleTime=-1
  To Workspace2 : ToWorkspace  VariableName=robot2_stateMeas  SaveFormat=Timeseries  SampleTime=-1
  To Workspace4 : ToWorkspace  VariableName=robot2_tauMeas  SaveFormat=Timeseries  SampleTime=-1
  To Workspace7 : ToWorkspace  Commented=on  VariableName=robot2_emergencyStop  SaveFormat=Timeseries  SampleTime=-1
  To Workspace9 : ToWorkspace  VariableName=robot2_trajCoMDes  SaveFormat=Timeseries  SampleTime=-1
  Torque Saturation : Saturate  Commented=on  UpperLimit=ConfigRobot2.Safety.torqueSaturation  LowerLimit=-ConfigRobot2.Safety.torqueSaturation
  emergency stop: joint limits1 : RobotStateLibrary/emergency stop: joint limits  Commented=on  Safety=ConfigRobot2.Safety
      settings: SourceProductName=robot-state-library
  state : Outport
  dynamics : Outport  Port=2
  link_state : Outport  Port=3
  L : Outport  Port=4
  wrench_Aeq : Outport  Port=5
  wrench_beq : Outport  Port=6
  wrench_Adeq : Outport  Port=7
  wrench_bdeq : Outport  Port=8
  tau_model : Outport  Port=9
  tau_sigma : Outport  Port=10
  link_state_ref : Outport  Port=11
  wires:
  GetMeasurement1/1 -> Postural Task Controller/4, Compute CoM Trajectory/5, Get Model State and Dynamics/3
  Get Model State and Dynamics/3 -> Momentum Controller/1, L/1
  Get Model State and Dynamics/1 -> Postural Task Controller/1, Momentum Controller/2, To Workspace2/1, state/1, State Yarp Publisher/1
  Get Model State and Dynamics/4 -> link_state/1, Momentum Controller/4, link_state_ref/1
  Get Model State and Dynamics/2 -> Postural Task Controller/2, Momentum Controller/5, dynamics/1
  Momentum Controller/3 -> wrench_Adeq/1
  Momentum Controller/4 -> wrench_bdeq/1
  Postural Task Controller/1 -> tau_model/1
  Postural Task Controller/2 -> tau_sigma/1
  Momentum Controller/1 -> wrench_Aeq/1
  Momentum Controller/2 -> wrench_beq/1
  tau/1 -> Torque Saturation/1
  GetMeasurement2/1 -> To Workspace4/1
  emergency stop: joint limits1/2 -> Bus Creator/2
  Bus Creator/1 -> To Workspace7/1
  emergency stop: joint limits1/3 -> Bus Creator/3
  emergency stop: joint limits1/1 -> Bus Creator/1
  Torque Saturation/1 -> emergency stop: joint limits1/2, To Workspace1/1, SetReferences/1
  Compute Base Transform from two links/1 -> ForwardKinematics/1
  GetMeasurement/1 -> emergency stop: joint limits1/1, Postural Task Controller/3, ForwardKinematics/2, Compute Base Transform from two links/2, Compute CoM Trajectory/1, Get Model State and Dynamics/2
  IdentityTransform2/1 -> Get Model State and Dynamics/1, Compute CoM Trajectory/4, Compute Base Transform from two links/1
  Compute CoM Trajectory/2 -> To Workspace9/1, Momentum Controller/3
  IdentityTransform3/1 -> Momentum Controller/6
  IdentityTransform4/1 -> Momentum Controller/7
  ForwardKinematics/1 -> "CoM6D -> CoMXYZ3"/1
  Constant/1 -> Compute CoM Trajectory/6, Compute CoM Trajectory/3
  "CoM6D -> CoMXYZ3"/1 -> Compute CoM Trajectory/2

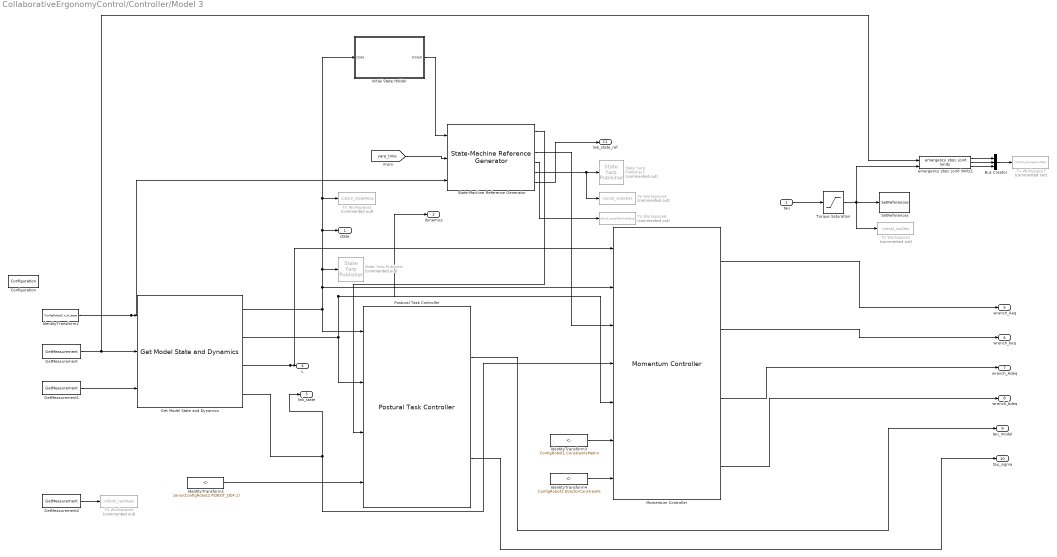
== system CollaborativeErgonomyControl/Controller/Model 3 ==
  tau : Inport
  Bus Creator : BusCreator  Inputs=3
  Configuration : WBToolboxLibrary/Utilities/Configuration  ConfigSource=Workspace  ConfigObject='WBTConfigRobot_2'  RobotName='icubSim'  UrdfFile='model.urdf'  ControlledJoints={'l_elbow','l_shoulder_pitch','torso_roll'}  ControlBoardsNames={'left_arm','right_arm','torso'}  LocalName='WBT'  GravityVector=[0,0,-9.81]
      settings: SourceProductName=WholeBodyToolbox
  Get Model State and Dynamics : RobotStateLibrary/Get Model State and Dynamics  nDoF=ConfigRobot2.ROBOT_DOF  regularization=0.001  contactFrame1Name=ConfigRobot2.Frames.LEFT_FOOT  contactFrame2Name=ConfigRobot2.Frames.RIGHT_FOOT  frame1=ConfigRobot2.Frames.LEFT_FOOT  frame2=ConfigRobot2.Frames.RIGHT_FOOT  frame3=ConfigRobot2.Frames.LEFT_HAND  frame4=ConfigRobot2.Frames.RIGHT_HAND
      settings: SourceProductName=robot-state-library
  GetMeasurement : WBToolboxLibrary/States/GetMeasurement  measuredType=Joints Position
      settings: SourceProductName=WholeBodyToolbox
  GetMeasurement1 : WBToolboxLibrary/States/GetMeasurement  measuredType=Joints Velocity
      settings: SourceProductName=WholeBodyToolbox
  GetMeasurement2 : WBToolboxLibrary/States/GetMeasurement  measuredType=Joints Torque
      settings: SourceProductName=WholeBodyToolbox
  IdentityTransform1 : Constant  Value=zeros(ConfigRobot2.ROBOT_DOF,1)
  IdentityTransform2 : Constant  Value=ConfigRobot2.w_H_base
  IdentityTransform3 : Constant  Value=ConfigRobot1.ConstraintsMatrix
  IdentityTransform4 : Constant  Value=ConfigRobot1.bVectorConstraints
  Initial State Holder : Subsystem
  Momentum Controller : RobotStateLibrary/Momentum Controller  GainMomentum=ConfigRobot2.Gains.GainMomentum  linksUseConstraintMatrix=ConfigRobot2.linksUseConstraintMatrix
      settings: SourceProductName=robot-state-library
  Postural Task Controller : RobotStateLibrary/Postural Task Controller  GainPostural=ConfigRobot2.Gains.GainPostural
      settings: SourceProductName=robot-state-library
  SetReferences : WBToolboxLibrary/Actuators/SetReferences  controlType=Torque  refSpeed=10*(pi/180)  refAcceleration=1000000*(pi/180)
      settings: SourceProductName=WholeBodyToolbox
  State Yarp Publisher : RobotStateLibrary/State Yarp Publisher  Commented=on  basePosePortName='/collaborativeController/robot2/basePose:o'  jointPosPortName='/collaborativeController/robot2/jointPosition:o'  nuPortName='/collaborativeController/robot2/stateVelocity:o'  posCoMPortName='/collaborativeController/robot2/CoMPosition:o'
      settings: SourceProductName=robot-state-library
  State Yarp Publisher1 : RobotStateLibrary/State Yarp Publisher  Commented=on  basePosePortName='/collaborativeController/robot2Ref/basePose:o'  jointPosPortName='/collaborativeController/robot2Ref/jointPosition:o'  nuPortName='/collaborativeController/robot2Ref/stateVelocity:o'  posCoMPortName='/collaborativeController/robot2Ref/CoMPosition:o'
      settings: SourceProductName=robot-state-library
  State-Machine Reference Generator : RobotStateLibrary/State-Machine Reference Generator  configStateMachine=ConfigRobot2.StateMachine  sampleTime=Config.tStep  frameName1=ConfigRobot2.Frames.LEFT_FOOT  frameName2=ConfigRobot2.Frames.RIGHT_FOOT  regularization=0.001  nDoF=ConfigRobot2.ROBOT_DOF  frame1=ConfigRobot2.Frames.LEFT_FOOT  frame2=ConfigRobot2.Frames.RIGHT_FOOT  frame3=ConfigRobot2.Frames.LEFT_HAND  frame4=ConfigRobot2.Frames.RIGHT_HAND
      settings: SourceProductName=robot-state-library
  To Workspace1 : ToWorkspace  Commented=on  VariableName=robot2_tauDes  SaveFormat=Timeseries  SampleTime=-1
  To Workspace2 : ToWorkspace  Commented=on  VariableName=robot2_stateMeas  SaveFormat=Timeseries  SampleTime=-1
  To Workspace3 : ToWorkspace  Commented=on  VariableName=robot2_stateDes  SaveFormat=Timeseries  SampleTime=-1
  To Workspace4 : ToWorkspace  Commented=on  VariableName=robot2_tauMeas  SaveFormat=Timeseries  SampleTime=-1
  To Workspace6 : ToWorkspace  Commented=on  VariableName=robot2_stateMachineState  SaveFormat=Timeseries  SampleTime=-1
  To Workspace7 : ToWorkspace  Commented=on  VariableName=robot2_emergencyStop  SaveFormat=Timeseries  SampleTime=-1
  Torque Saturation : Saturate  UpperLimit=ConfigRobot2.Safety.torqueSaturation  LowerLimit=-ConfigRobot2.Safety.torqueSaturation
  emergency stop: joint limits1 : RobotStateLibrary/emergency stop: joint limits  Safety=ConfigRobot2.Safety
      settings: SourceProductName=robot-state-library
  state : Outport
  dynamics : Outport  Port=2
  link_state : Outport  Port=3
  L : Outport  Port=4
  wrench_Aeq : Outport  Port=5
  wrench_beq : Outport  Port=6
  wrench_Adeq : Outport  Port=7
  wrench_bdeq : Outport  Port=8
  tau_model : Outport  Port=9
  tau_sigma : Outport  Port=10
  link_state_ref : Outport  Port=11
  wires:
  IdentityTransform1/1 -> Postural Task Controller/4
  GetMeasurement/1 -> emergency stop: joint limits1/1, Get Model State and Dynamics/2
  GetMeasurement1/1 -> Get Model State and Dynamics/3
  IdentityTransform2/1 -> State-Machine Reference Generator/3, Get Model State and Dynamics/1
  Get Model State and Dynamics/3 -> Momentum Controller/1, L/1
  State-Machine Reference Generator/3 -> Momentum Controller/3
  IdentityTransform3/1 -> Momentum Controller/6
  IdentityTransform4/1 -> Momentum Controller/7
  [yarp_time] -> State-Machine Reference Generator/2
  State-Machine Reference Generator/1 -> Postural Task Controller/3
  State-Machine Reference Generator/5 -> To Workspace3/1, State Yarp Publisher1/1
  Get Model State and Dynamics/1 -> Postural Task Controller/1, Momentum Controller/2, To Workspace2/1, Initial State Holder/1(state), state/1, State Yarp Publisher/1
  Initial State Holder/1(state0) -> State-Machine Reference Generator/1
  Get Model State and Dynamics/4 -> link_state/1, Momentum Controller/4
  Get Model State and Dynamics/2 -> Postural Task Controller/2, Momentum Controller/5, dynamics/1
  Momentum Controller/3 -> wrench_Adeq/1
  Momentum Controller/4 -> wrench_bdeq/1
  Postural Task Controller/1 -> tau_model/1
  Postural Task Controller/2 -> tau_sigma/1
  Momentum Controller/1 -> wrench_Aeq/1
  Momentum Controller/2 -> wrench_beq/1
  State-Machine Reference Generator/6 -> link_state_ref/1
  tau/1 -> Torque Saturation/1
  GetMeasurement2/1 -> To Workspace4/1
  emergency stop: joint limits1/2 -> Bus Creator/2
  Bus Creator/1 -> To Workspace7/1
  emergency stop: joint limits1/3 -> Bus Creator/3
  emergency stop: joint limits1/1 -> Bus Creator/1
  State-Machine Reference Generator/4 -> To Workspace6/1
  Torque Saturation/1 -> emergency stop: joint limits1/2, To Workspace1/1, SetReferences/1
